simulink model "hinta"  (Simulink 7.8)
settings: Solver=ode45  StartTime=0.0  StopTime=100  RelTol=1e-3
libraries: vrlib x3, simulink x1
settings Model: Creator=valaki  LastModifiedBy=valaki

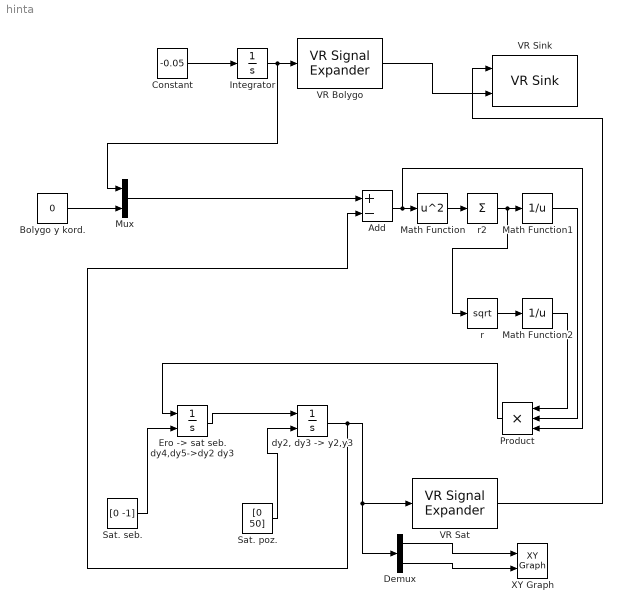
== system hinta ==
  Add : Sum  Inputs=+-
  Bolygo y kord. : Constant  Value=0
  Constant : Constant  Value=-0.05
  Demux : Demux  Outputs=2
  "Ero -> sat seb. dy4,dy5->dy2 dy3" : Integrator  InitialConditionSource=external
  Integrator : Integrator
  Math Function : Math  Operator=square  SaturateOnIntegerOverflow=on
  Math Function1 : Math  Operator=reciprocal  SaturateOnIntegerOverflow=on
  Math Function2 : Math  Operator=reciprocal  SaturateOnIntegerOverflow=on
  Mux : Mux  Inputs=2
  Product : Product  Inputs=3  RndMeth=Zero
  Sat. poz. : Constant  Value=[0 50]
  Sat. seb. : Constant  Value=[0 -1]
  VR Bolygo : vrlib/VR Signal Expander  outwidth=3  outidx=[1]
  VR Sat : vrlib/VR Signal Expander  outwidth=3  outidx=[1 2]
  VR Sink : vrlib/VR Sink  SampleTime=0.1  ViewEnable=on  RemoteChange=off  RemoteView=off  FieldsWritten=Satellite.translation.3.1.1.double#Luminary.translation.3.1.1.double  WorldFileName=satellite.wrl  AutoView=off  VideoDimensions=[]  AllowVariableSize=off  FigureProperties="{'Position', 'Name', 'Viewpoint', 'CameraBound', 'CameraDirection', 'CameraPosition', 'CameraUpVector', 'ZoomFactor', 'Antialiasing', 'Headlight', 'Lighting', 'NavPanel', 'StatusBar', 'ToolBar', 'Textures', 'Transparency', 'Triad', 'Wireframe', 'NavZones', 'NavMode', 'NavSpeed', 'CaptureFileFormat', 'CaptureFileName', 'Record2DCompressMethod', 'Record2DCompressQuality', 'Record2D', 'Record2DFileName', 'Record2DFPS'; [5.0000000000000000e+000  9.2000000000000000e+001  5.7600000000000000e+002  3.8000000000000000e+002], '', 'Ball', 'on', [0.0000000000000000e+000  0.0000000000000000e+000 -1.0000000000000000e+000], [0.0000000000000000e+000  0.0000000000000000e+000  6.4000000000000000e+001], [0.0000000000000000e+000  1.0000000000000000e+000  0.0000000000000000e+000], [1.0000000000000000e+000], 'on', 'on', 'on', 'halfbar', 'on', 'on', 'on', 'on', 'none', 'off', 'off', 'fly', 'normal', 'tif', '%f_anim_%n.tif', 'auto', [7.5000000000000000e+001], 'off', '%f_anim_%n.avi', [1.5000000000000000e+001]}"
  XY Graph : simulink/Sinks/XY Graph  xmin=-50  xmax=50  ymin=-50  ymax=50  st=-1
  "dy2, dy3 -> y2,y3" : Integrator  InitialConditionSource=external
  r : Sqrt  SaturateOnIntegerOverflow=on
  r2 : Sum  Inputs=+
  wires:
  Constant/1 -> Integrator/1
  Integrator/1 -> VR Bolygo/1, Mux/1
  VR Bolygo/1 -> VR Sink/2
  Bolygo y kord./1 -> Mux/2
  "Ero -> sat seb. dy4,dy5->dy2 dy3"/1 -> "dy2, dy3 -> y2,y3"/1
  Sat. seb./1 -> "Ero -> sat seb. dy4,dy5->dy2 dy3"/2
  Sat. poz./1 -> "dy2, dy3 -> y2,y3"/2
  VR Sat/1 -> VR Sink/1
  "dy2, dy3 -> y2,y3"/1 -> Add/2, VR Sat/1, Demux/1
  Mux/1 -> Add/1
  Add/1 -> Math Function/1, Product/3
  Math Function/1 -> r2/1
  r2/1 -> Math Function1/1, r/1
  r/1 -> Math Function2/1
  Product/1 -> "Ero -> sat seb. dy4,dy5->dy2 dy3"/1
  Math Function2/1 -> Product/1
  Math Function1/1 -> Product/2
  Demux/1 -> XY Graph/1
  Demux/2 -> XY Graph/2
